simulink model "OperationalSpaceGravityCompensation"  (R2022b)
settings: Solver=VariableStepAuto  StartTime=0.0  StopTime=5  RelTol=1e-3
values from neighbouring files (symbols this model uses):
  Kd = diag([230,230,230,1,1,1])    [parameters.m]
  Kp = diag([500,500,500,3,3,3])    [parameters.m]
  xd = [H(1:3,4); eulers']    [parameters.m]
settings Model: Creator=uzair  LastModifiedBy=uzair

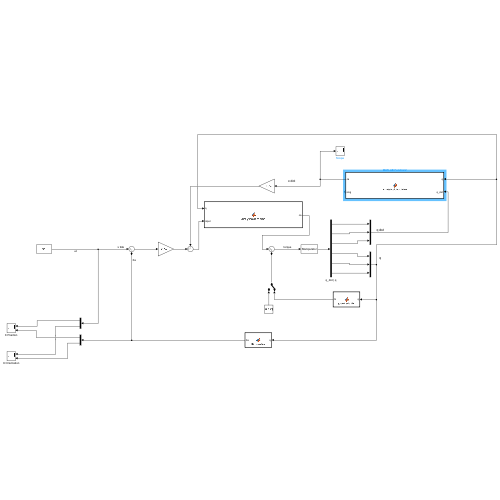
[thumbnail: Simulink's stored preview of the top-level diagram]
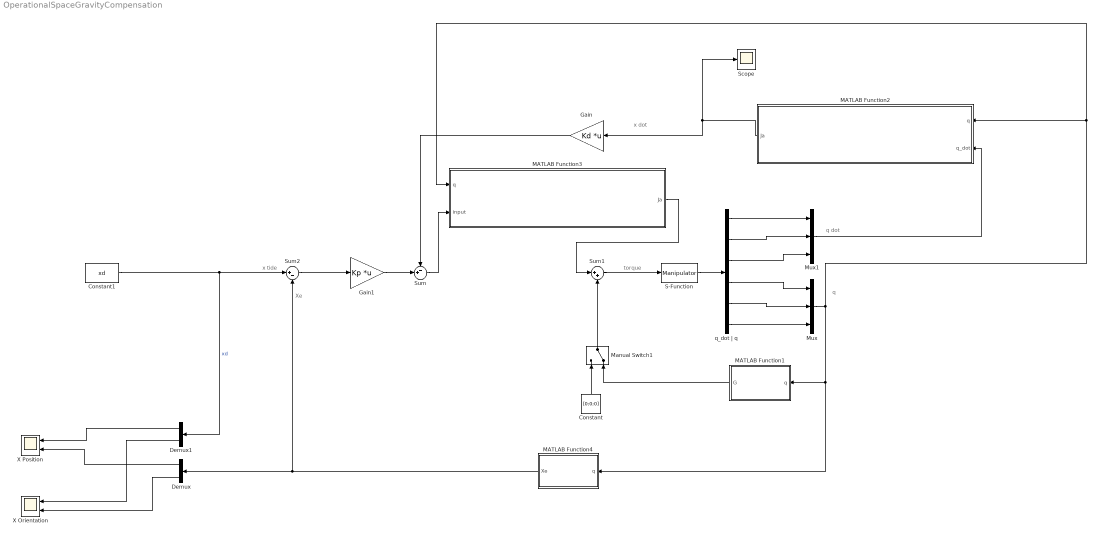
== system OperationalSpaceGravityCompensation ==
  note: torque
  note: x tide
  note: q
  note: q dot
  note: Xe
  note: x dot
  Constant : Constant  Value=[0;0;0]
  Constant1 : Constant  Value=xd
  Demux : Demux  Outputs=2
  Demux1 : Demux  Outputs=2
  Gain : Gain  Gain=Kd  Multiplication=Matrix(K*u)
  Gain1 : Gain  Gain=Kp  Multiplication=Matrix(K*u)
  MATLAB Function1 : MATLAB Function  TreatAsAtomicUnit=on
  MATLAB Function2 : MATLAB Function  TreatAsAtomicUnit=on
  MATLAB Function3 : MATLAB Function  TreatAsAtomicUnit=on
  MATLAB Function4 : MATLAB Function  TreatAsAtomicUnit=on
  Manual Switch1 : ManualSwitch  CurrentSetting=0
  Mux : Mux  Inputs=3
  Mux1 : Mux  Inputs=3
  S-Function : S-Function  FunctionName=Manipulator  Parameters=params  SFunctionDeploymentMode=off  EnableBusSupport=off
  Scope : Scope
  Sum : Sum  Inputs=-+|
  Sum1 : Sum  Inputs=|++
  Sum2 : Sum  Inputs=|+-
  X Orientation : Scope  NumInputPorts=2
  X Position : Scope  NumInputPorts=2
  q_dot | q : Demux  Outputs=6
  wires:
  S-Function/1 -> q_dot | q/1
  q_dot | q/6 -> Mux/3
  q_dot | q/5 -> Mux/2
  q_dot | q/4 -> Mux/1
  q_dot | q/1 -> Mux1/1
  q_dot | q/2 -> Mux1/2
  q_dot | q/3 -> Mux1/3
  Gain/1 -> Sum/1
  Sum1/1 -> S-Function/1
  Mux/1 -> MATLAB Function2/1(q), MATLAB Function3/1(q), MATLAB Function1/1(q), MATLAB Function4/1(q)
  Gain1/1 -> Sum/2
  Sum2/1 -> Gain1/1
  MATLAB Function1/1(G) -> Manual Switch1/2
  Constant/1 -> Manual Switch1/1
  Mux1/1 -> MATLAB Function2/2(q_dot)
  MATLAB Function4/1(Xe) -> Demux/1, Sum2/2
  Constant1/1 -> Demux1/1, Sum2/1  "xd"
  Demux1/1 -> X Position/1
  Demux/1 -> X Position/2
  Demux1/2 -> X Orientation/1
  Demux/2 -> X Orientation/2
  MATLAB Function2/1(Ja) -> Gain/1, Scope/1
  Manual Switch1/1 -> Sum1/2
  MATLAB Function3/1(Ja) -> Sum1/1
  Sum/1 -> MATLAB Function3/2(input)

== matlab function OperationalSpaceGravityCompensation/MATLAB Function1 ==
  data: q input; G output; params parameter
function G = gravityMatrix(q, params)
    q1 = q(1);
    q2 = q(2);
    q3 = q(3);
    
    g = params.g;

    m1 = params.m(1);
    m2 = params.m(2);
    m3 = params.m(3);

    G = [(g*m1*cos(q1))/5 - g*m2*((3*sin(q1))/20 - (2*cos(q1))/5 + q2*sin(q1)) + g*m3*((2*cos(q1))/5 + (2*cos(q1)*cos(q3))/25 - sin(q1)*(q2 + 3/10));
                                                                                                                        g*cos(q1)*(m2 + m3);
                                                                                                               -(2*g*m3*sin(q1)*sin(q3))/25];
end

== matlab function OperationalSpaceGravityCompensation/MATLAB Function3 ==
  data: q input; Ja output; input input
function Ja = AnalyticalJacobian(q,input)
    q1 = q(1);
    q2 = q(2);
    q3 = q(3);

    H = [[ sin(q1), -cos(q1)*sin(q3), cos(q1)*cos(q3), (2*cos(q1))/5 + (4*cos(q1)*cos(q3))/25 - sin(q1)*(q2 + 3/10)]
[-cos(q1), -sin(q1)*sin(q3), cos(q3)*sin(q1), (2*sin(q1))/5 + cos(q1)*(q2 + 3/10) + (4*cos(q3)*sin(q1))/25]
[       0,         -cos(q3),        -sin(q3),                                              -(4*sin(q3))/25]
[       0,                0,               0,                                                            1]];


eulers = rotm2eul(H(1:3,1:3), "ZYZ");


    phi1 = eulers(1);
    phi2 = eulers(2);
    phi3 = eulers(3); %not used

Ja_m = [
[- (2*sin(q1))/5 - cos(q1)*(q2 + 3/10) - (4*cos(q3)*sin(q1))/25, -sin(q1),               -(4*cos(q1)*sin(q3))/25]
[  (2*cos(q1))/5 + (4*cos(q1)*cos(q3))/25 - sin(q1)*(q2 + 3/10),  cos(q1),               -(4*sin(q1)*sin(q3))/25]
[                                                             0,        0,                       -(4*cos(q3))/25]
[                                                             1,        0, -(sin(phi1 - q1)*cos(phi2))/sin(phi2)]
[                                                             0,        0,                        cos(phi1 - q1)]
[                                                             0,        0,              sin(phi1 - q1)/sin(phi2)]
];


    Ja = Ja_m' *input;
end

== matlab function OperationalSpaceGravityCompensation/MATLAB Function2 ==
  data: q input; Ja output; q_dot input
function Ja = AnalyticalJacobian(q,q_dot)
    q1 = q(1);
    q2 = q(2);
    q3 = q(3);

    H = [[ sin(q1), -cos(q1)*sin(q3), cos(q1)*cos(q3), (2*cos(q1))/5 + (4*cos(q1)*cos(q3))/25 - sin(q1)*(q2 + 3/10)]
[-cos(q1), -sin(q1)*sin(q3), cos(q3)*sin(q1), (2*sin(q1))/5 + cos(q1)*(q2 + 3/10) + (4*cos(q3)*sin(q1))/25]
[       0,         -cos(q3),        -sin(q3),                                              -(4*sin(q3))/25]
[       0,                0,               0,                                                            1]];


eulers = rotm2eul(H(1:3,1:3), "ZYZ");


    phi1 = eulers(1);
    phi2 = eulers(2);
    phi3 = eulers(3); %not used

Ja_m = [
[- (2*sin(q1))/5 - cos(q1)*(q2 + 3/10) - (4*cos(q3)*sin(q1))/25, -sin(q1),               -(4*cos(q1)*sin(q3))/25]
[  (2*cos(q1))/5 + (4*cos(q1)*cos(q3))/25 - sin(q1)*(q2 + 3/10),  cos(q1),               -(4*sin(q1)*sin(q3))/25]
[                                                             0,        0,                       -(4*cos(q3))/25]
[                                                             1,        0, -(sin(phi1 - q1)*cos(phi2))/sin(phi2)]
[                                                             0,        0,                        cos(phi1 - q1)]
[                                                             0,        0,              sin(phi1 - q1)/sin(phi2)]
];


    Ja = Ja_m * q_dot;
end

== matlab function OperationalSpaceGravityCompensation/MATLAB Function4 ==
  data: q input; Xe output
function Xe = Kinematics(q)
    q1 = q(1);
    q2 = q(2);
    q3 = q(3);
    
    H = [[ sin(q1), -cos(q1)*sin(q3), cos(q1)*cos(q3), (2*cos(q1))/5 + (4*cos(q1)*cos(q3))/25 - sin(q1)*(q2 + 3/10)]
[-cos(q1), -sin(q1)*sin(q3), cos(q3)*sin(q1), (2*sin(q1))/5 + cos(q1)*(q2 + 3/10) + (4*cos(q3)*sin(q1))/25]
[       0,         -cos(q3),        -sin(q3),                                              -(4*sin(q3))/25]
[       0,                0,               0,                                                            1]];

    eulers = rotm2eul(H(1:3,1:3), "ZYZ");

    Xe = [H(1:3,4); eulers'];
end
